simulink model "labo3parte1"  (R2025b)
settings: Solver=FixedStepAuto  StartTime=0.0  StopTime=60  RelTol=1e-3  EnableMultiTasking=on
values from neighbouring files (symbols this model uses):
  Ts = 0.1    [Labo2_Datos.mat]
undefined symbols (not defined in the file or in its folder): sys, sysd
libraries: arduinolib x3, eeLuenbergerObserver x2, arduinosensorlib x1
settings Model: ExtModeTrigDuration=2  Creator=ALIENWARE-GAMER  LastModifiedBy=Froilán Pardo
settings SolverCC: AutoInsertRateTranBlk=on
settings OptimizationCC: BlockReduction=off  BooleanDataType=off  EnhancedBackFolding=on  PassReuseOutputArgsAs=Individual arguments  ZeroExternalMemoryAtStartup=off  ZeroInternalMemoryAtStartup=off  MaxStackSize=64  OptimizeBlockOrder=speed  DifferentSizesBufferReuse=on  OptimizationCustomize=off  EfficientTunableParamExpr=on
settings DebuggingCC: SaveWithParameterizedLinksMsg=none  UnderspecifiedInitializationDetection=Classic  MergeDetectMultiDrivingBlocksExec=none  SignalResolutionControl=TryResolveAllWithWarning  ParameterTunabilityLossMsg=error
settings HardwareCC: ProdBitPerInt=16.0  ProdBitPerPointer=16.0  ProdBitPerSizeT=16.0  ProdBitPerPtrDiffT=16.0  ProdLargestAtomicFloat=None  ProdWordSize=8.0  ProdHWDeviceType=Atmel->AVR  TargetBitPerInt=16.0  TargetBitPerPointer=16.0  TargetBitPerSizeT=16.0  TargetBitPerPtrDiffT=16.0  TargetIntDivRoundTo=Zero  TargetEndianess=LittleEndian  TargetWordSize=8.0  TargetHWDeviceType=Atmel->AVR
settings ModelReferenceCC: PropagateSignalLabelsOutOfModel=off
settings SFSimCC: MATLABDynamicMemAlloc=off
settings RTWCC: SystemTargetFile=ert.tlc  HardwareBoard=Arduino Uno  TemplateMakefile=ert_default_tmf  Toolchain=Arduino AVR  BuildConfiguration=Faster Runs  Description=Embedded Coder
settings CodeAppCC: ForceParamTrailComments=on  IgnoreCustomStorageClasses=off  OperatorAnnotations=on  SimulinkDataObjDesc=on  SFDataObjDesc=on  InsertBlockDesc=on
settings ERTTargetCC: ExtModeTransport=3.0  ExtModeStaticAlloc=on  ExtModeAutomaticAllocSize=off  ExtModeStaticAllocSize=250.0  ExtModeMexFile=ext_xcp  ExtModeIntrfLevel=Level2 - Open  InlinedParameterPlacement=Hierarchical  SupportContinuousTime=on  SupportVariableSizeSignals=on

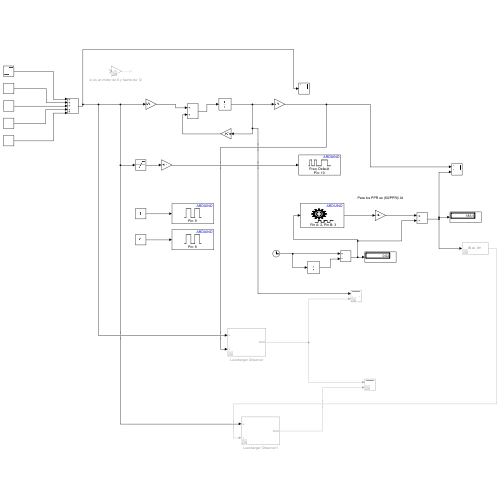
[thumbnail: Simulink's stored preview of the top-level diagram]
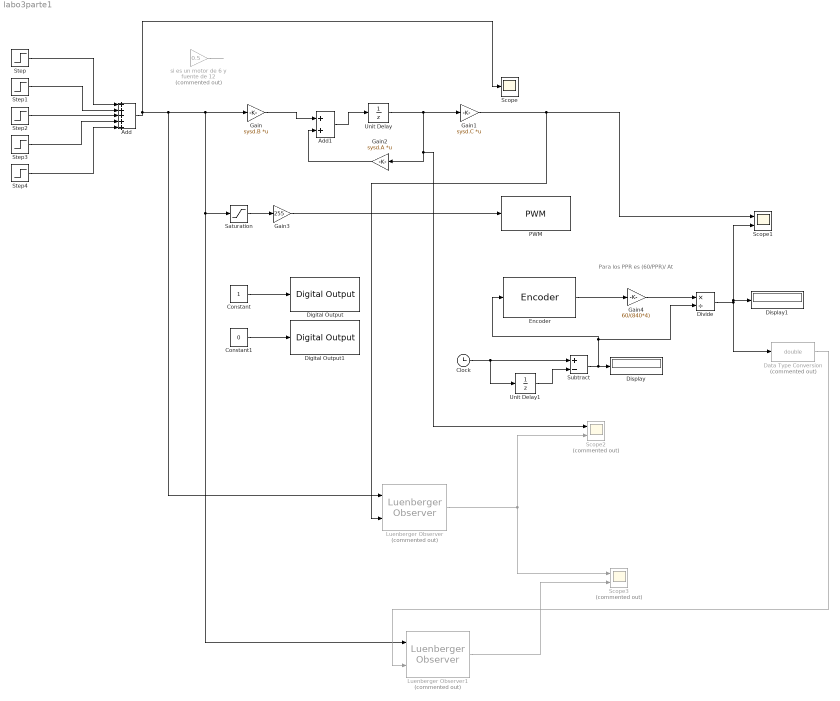
== system labo3parte1 ==
  note: Para los PPR es (60/PPR)/ At
  Add : Sum  Inputs=+++++
  Add1 : Sum
  Clock : Clock
  Constant : Constant
  Constant1 : Constant  Value=0
  Data Type Conversion : DataTypeConversion  Commented=on  OutDataTypeStr=double  SaturateOnIntegerOverflow=off  RndMeth=Floor
  Digital Output : arduinolib/Digital Output  pinNumber=9  Direction=output  blockPlatform=arduino
  Digital Output1 : arduinolib/Digital Output  pinNumber=8  Direction=output  blockPlatform=arduino
  Display : Display
  Display1 : Display
  Divide : Product  Inputs=*/
  Encoder : arduinosensorlib/Encoder  InputA=2  InputB=3  Mode=Reset by external signal  SampleTime=-1
  Gain : Gain  Gain=sysd.B  Multiplication=Matrix(K*u)
  Gain1 : Gain  Gain=sysd.C  Multiplication=Matrix(K*u)
  Gain2 : Gain  Gain=sysd.A  Multiplication=Matrix(K*u)
  Gain3 : Gain  Gain=255
  Gain4 : Gain  Gain=60/(840*4)
  Luenberger Observer : eeLuenbergerObserver/Luenberger Observer  Commented=on  StateSpaceType=Discrete-time  Ad=sysd.A  Bd=sysd.B  Cd=sysd.C  Dd=sysd.D  A=1  B=1  C=1  D=1  ObserverDesign=Desired eigenvalues  Ld=1  DesiredEigenvalues=exp(eig(sys.A)*Ts)  x0=[0;0]  Tsd=0.1  Ts=0.1
      settings: LibrarySourceBlock=ee_sl_lib/Observers/Luenberger Observer
  Luenberger Observer1 : eeLuenbergerObserver/Luenberger Observer  Commented=on  StateSpaceType=Discrete-time  Ad=sysd.A  Bd=sysd.B  Cd=sysd.C  Dd=sysd.D  A=1  B=1  C=1  D=1  ObserverDesign=Desired eigenvalues  Ld=1  DesiredEigenvalues=exp(5*eig(sys.A)*Ts)  x0=[0;0]  Tsd=0.1  Ts=0.1
      settings: LibrarySourceBlock=ee_sl_lib/Observers/Luenberger Observer
  PWM : arduinolib/PWM  pinNumber=10  frequencyType=Default  desiredFrequency=490.2  achievableFrequency=490.2
  Saturation : Saturate  UpperLimit=1  LowerLimit=0
  Scope : Scope
      settings: ActiveDisplayYMinimum=0.10000000000000003  ActiveDisplayYMaximum=1.1
  Scope1 : Scope  NumInputPorts=2
      settings: ActiveDisplayYMinimum=-3.4718852156771182E+37  ActiveDisplayYMaximum=3.1010626004731196E+38
  Scope2 : Scope  Commented=on  NumInputPorts=2
      settings: ActiveDisplayYMinimum=-200.17917061901909  ActiveDisplayYMaximum=1791.2427535332395  DataLoggingVariableName=ScopeData2
  Scope3 : Scope  Commented=on  NumInputPorts=2
      settings: ActiveDisplayYMinimum=-1  ActiveDisplayYMaximum=1  DataLoggingVariableName=ScopeData3
  Step : Step  Time=0  After=0.2  SampleTime=0
  Step1 : Step  Time=12  After=0.2  SampleTime=0
  Step2 : Step  Time=24  After=0.2  SampleTime=0
  Step3 : Step  Time=36  After=0.2  SampleTime=0
  Step4 : Step  Time=48  After=0.2  SampleTime=0
  Subtract : Sum  Inputs=+-
  Unit Delay : UnitDelay  SampleTime=Ts  HasFrameUpgradeWarning=on
  Unit Delay1 : UnitDelay  SampleTime=-1  HasFrameUpgradeWarning=on
  "si es un motor de 6 y fuente de 12 " : Gain  Commented=on  Gain=0.5
  wires:
  Step/1 -> Add/1
  Step1/1 -> Add/2
  Step2/1 -> Add/3
  Step3/1 -> Add/4
  Step4/1 -> Add/5
  Add/1 -> Scope/1, Luenberger Observer1/1, Saturation/1, Gain/1, Luenberger Observer/1
  "si es un motor de 6 y fuente de 12 "/1 -> ?
  Gain/1 -> Add1/1
  Add1/1 -> Unit Delay/1
  Gain2/1 -> Add1/2
  Unit Delay/1 -> Scope2/1, Gain2/1, Gain1/1
  Gain1/1 -> Luenberger Observer/2, Scope1/1
  Constant/1 -> Digital Output/1
  Constant1/1 -> Digital Output1/1
  Gain3/1 -> PWM/1
  Saturation/1 -> Gain3/1
  Clock/1 -> Unit Delay1/1, Subtract/1
  Unit Delay1/1 -> Subtract/2
  Subtract/1 -> Divide/2, Encoder/1, Display/1
  Encoder/1 -> Gain4/1
  Gain4/1 -> Divide/1
  Divide/1 -> Display1/1, Scope1/2, Data Type Conversion/1
  Luenberger Observer/1 -> Scope2/2, Scope3/1
  Luenberger Observer1/1 -> Scope3/2
  Data Type Conversion/1 -> Luenberger Observer1/2
